simulink model "RS"  (Simulink 3.00)
settings: Solver=ode45  StartTime=0.0  StopTime=10.0  RelTol=1e-3
settings Model: AlgebraicLoopMsg=none  InheritedTsInSrcMsg=none

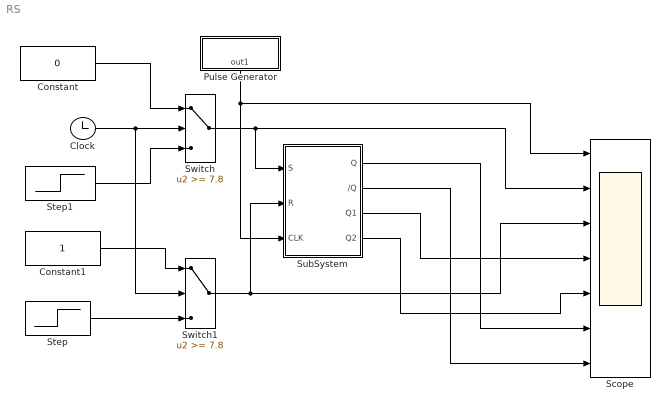
== system RS ==
  Clock : Clock
      settings: DisplayTime=off  Decimation=10
  Constant : Constant  Value=0
  Constant1 : Constant  Value=1
  Pulse Generator : Subsystem  Orientation=down  mask(Pulse Generator){period=1, duty=50, amplitude=1, start=0}
      mask prompts: period "Period (secs):"; duty "Duty cycle (% of period):"; start "Start time:"
      mask help: Pulse Generator
      mask Help: Pulse generator which ensures pulse transitions are hit. Provides a vector of pulses when the height is entered as a vector.  Unmask to see how it works.
      mask Display: plot(0,0,100,100,[95,90,90,75,75,60,60,45,45,30,30,15,15,5],[25,25,75,75,25,25,75,75,25,25,75,75,25,25]);
  Scope : Scope  NumInputPorts=7
      settings: TickLabels=on  TimeRange=10  YMin=0~0~0~0~0~0~0  YMax=1.2~1.2~1.2~1.2~1.2~1.2~1.2  SaveToWorkspace=off  SaveName=ScopeData
  Step : Step  Time=4.2  Before=1  After=0  SampleTime=-1
  Step1 : Step  Time=4.2  Before=0  After=1  SampleTime=-1
  SubSystem : Subsystem
  Switch : Switch  Threshold=7.8
  Switch1 : Switch  Threshold=7.8
  wires:
  Step1/1 -> Switch/3
  Step/1 -> Switch1/3
  Clock/1 -> Switch/2, Switch1/2
  Pulse Generator/1(out1) -> Scope/1, SubSystem/3(CLK)
  Switch/1 -> SubSystem/1(S), Scope/2
  Switch1/1 -> SubSystem/2(R), Scope/3
  SubSystem/3(Q1) -> Scope/4
  SubSystem/4(Q2) -> Scope/5
  SubSystem/1(Q) -> Scope/6
  SubSystem/2(/Q) -> Scope/7
  Constant/1 -> Switch/1
  Constant1/1 -> Switch1/1

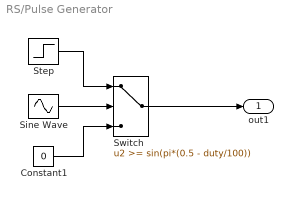
== system RS/Pulse Generator ==
  Constant1 : Constant  Value=0
  Sine Wave : Sin  Amplitude=1  Frequency=2*pi./period  Phase=-2*pi*(start./period + duty/200 - 1/4)  SampleTime=-1
  Step : Step  Time=start  Before=0  After=amplitude  SampleTime=-1
  Switch : Switch  Threshold=sin(pi*(0.5 - duty/100))
  out1 : Outport  Port=1  InitialOutput=0
  wires:
  Sine Wave/1 -> Switch/2
  Switch/1 -> out1/1
  Constant1/1 -> Switch/3
  Step/1 -> Switch/1

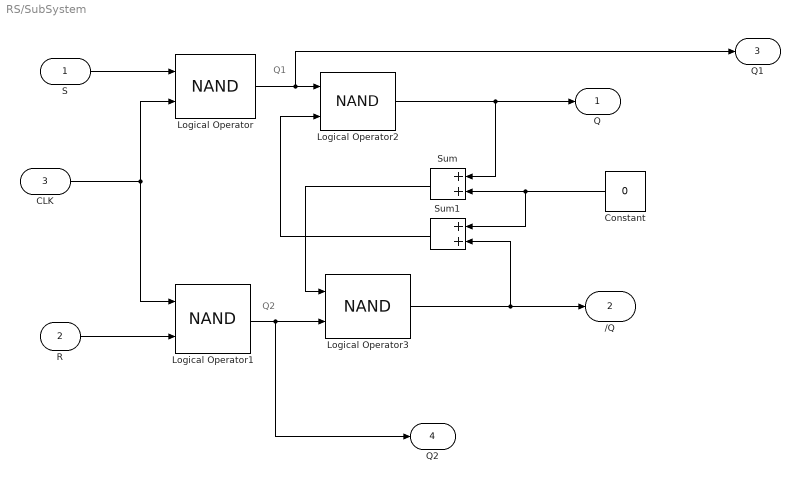
== system RS/SubSystem ==
  note: Q1
  note: Q2
  S : Inport  Port=1  PortWidth=-1  SampleTime=-1  DataType=auto
      settings: SignalType=auto
  R : Inport  Port=2  PortWidth=-1  SampleTime=-1  DataType=auto
      settings: SignalType=auto
  CLK : Inport  Port=3  PortWidth=-1  SampleTime=-1  DataType=auto
      settings: SignalType=auto
  Constant : Constant  Orientation=left  Value=0
  Logical Operator{,1..3} (4 alike) : Logic  Operator=NAND  Inputs=2
  Sum : Sum  Orientation=left  Inputs=++  SaturateOnIntegerOverflow=on
  Sum1 : Sum  Orientation=left  Inputs=++  SaturateOnIntegerOverflow=on
  Q : Outport  Port=1
  /Q : Outport  Port=2
  Q1 : Outport  Port=3
  Q2 : Outport  Port=4
  wires:
  S/1 -> Logical Operator/1
  CLK/1 -> Logical Operator1/1, Logical Operator/2
  R/1 -> Logical Operator1/2
  Logical Operator1/1 -> Logical Operator3/2, Q2/1
  Logical Operator/1 -> Logical Operator2/1, Q1/1
  Logical Operator2/1 -> Q/1, Sum/1
  Sum/1 -> Logical Operator3/1
  Logical Operator3/1 -> /Q/1, Sum1/2
  Sum1/1 -> Logical Operator2/2
  Constant/1 -> Sum1/1, Sum/2
